simulink model "ep1_3"  (R2018a)
settings: Solver=VariableStepAuto  StartTime=0.0  StopTime=10.0  RelTol=1e-3
settings Model: Creator=zheny  LastModifiedBy=zheny

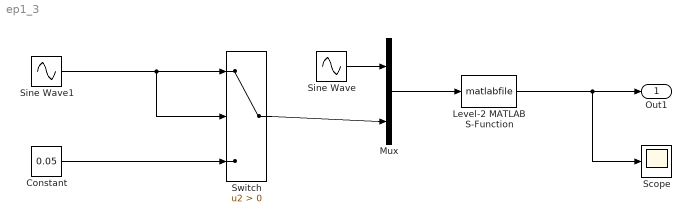
== system ep1_3 ==
  Constant : Constant  Value=0.05
  Level-2 MATLAB S-Function : M-S-Function
  Mux : Mux  Inputs=2
  Scope : Scope
  Sine Wave : Sin  SampleTime=0
  Sine Wave1 : Sin  SampleTime=0
  Switch : Switch  Criteria=u2 > Threshold
  Out1 : Outport
  wires:
  Sine Wave1/1 -> Switch/2, Switch/1
  Constant/1 -> Switch/3
  Switch/1 -> Mux/2
  Sine Wave/1 -> Mux/1
  Mux/1 -> Level-2 MATLAB S-Function/1
  Level-2 MATLAB S-Function/1 -> Out1/1, Scope/1
